simulink model "sgMdl_ResistorEmulation"  (R2024b)
settings: Solver=FixedStepAuto  StartTime=0.0  StopTime=inf  RelTol=1e-3  EnableMultiTasking=on
libraries: speedgoatlib_PIL x1, simulink x1
Description:
  | Resistor Emulation
settings Model: ModifiedByFormat=Speedgoat  SimulationMode=external  ExtModeTrigDuration=100000  Creator=Speedgoat  LastModifiedBy=Speedgoat
settings SolverCC: ConcurrentTasks=on  AlgebraicLoopSolver=TrustRegion  PositivePriorityOrder=on  InsertRTBMode=Never (minimum delay)
settings DataIOCC: SaveFormat=Array  SaveState=on  SignalLoggingName=logsOut
settings OptimizationCC: BlockReduction=off  BooleanDataType=off  OptimizeBlockIOStorage=off  BufferReuse=off  ReuseModelBlockBuffer=off  GlobalBufferReuse=off  ExpressionFolding=off  LocalBlockOutputs=off  InitFltsAndDblsToZero=on  OptimizeDataStoreBuffers=off  BusAssignmentInplaceUpdate=off
settings DebuggingCC: SaveWithParameterizedLinksMsg=none  UnderspecifiedInitializationDetection=Classic  MergeDetectMultiDrivingBlocksExec=none  CheckExecutionContextPreStartOutputMsg=on  SignalResolutionControl=TryResolveAllWithWarning  TasksWithSamePriorityMsg=none  UnconnectedInputMsg=warning  UnconnectedOutputMsg=warning  UnconnectedLineMsg=warning  SFUnexpectedBacktrackingDiag=warning  SFNoUnconditionalDefaultTransitionDiag=warning  SFExecutionAtInitializationDiag=none  ArithmeticOperatorsInVariantConditions=warning
settings HardwareCC: ProdBitPerLong=64  ProdLongLongMode=on  ProdHWDeviceType=Intel->x86-64 (Linux 64)
settings ModelReferenceCC: EnableRefExpFcnMdlSchedulingChecks=on  PropagateSignalLabelsOutOfModel=off
settings SFSimCC: SimUseLocalCustomCode=off  SimTargetLang=C++
settings RTWCC: Description=Speedgoat Real-Time Target Machine  SystemTargetFile=speedgoat.tlc  TemplateMakefile=slrealtime_default_tmf  PostCodeGenCommand=sg.model.build.makeCfg(bdroot, buildInfo);  RTWUseLocalCustomCode=off  Toolchain=Simulink Real-Time Toolchain  BuildConfiguration=Faster Runs  TargetLang=C++  GPUComputeCapability=3.5  DLArmComputeVersion=19.05
settings CodeAppCC: StateflowObjectComments=on
settings SimulinkRealTimeTargetCC: SubcomponentCodeInterfacePackaging=Reusable function  MATLABClassNameForMDSCustomization=Simulink.SoftwareTarget.GRTCustomization  InstructionSetFMA=off  LogToMDFFile=off  SLRTFileLogMaxRuns=10  UseGCCFastMath=on
settings ConfigComp: CovMetricSettings=dw  CovSaveCumulativeToWorkspaceVar=on  CovSaveSingleToWorkspaceVar=on  CovExternalEMLEnable=off  CovSFcnEnable=off  CovBoundaryAbsTol=1.0e-5

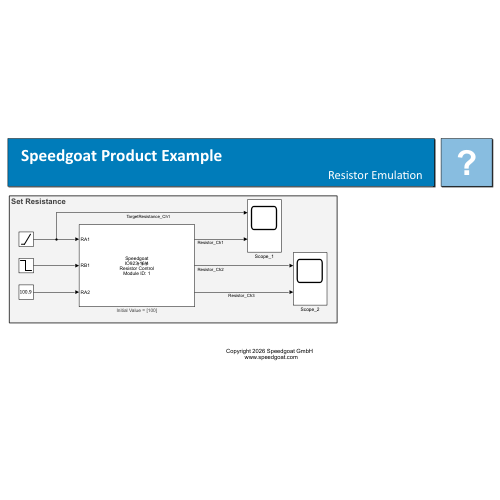
[thumbnail: Simulink's stored preview of the top-level diagram]
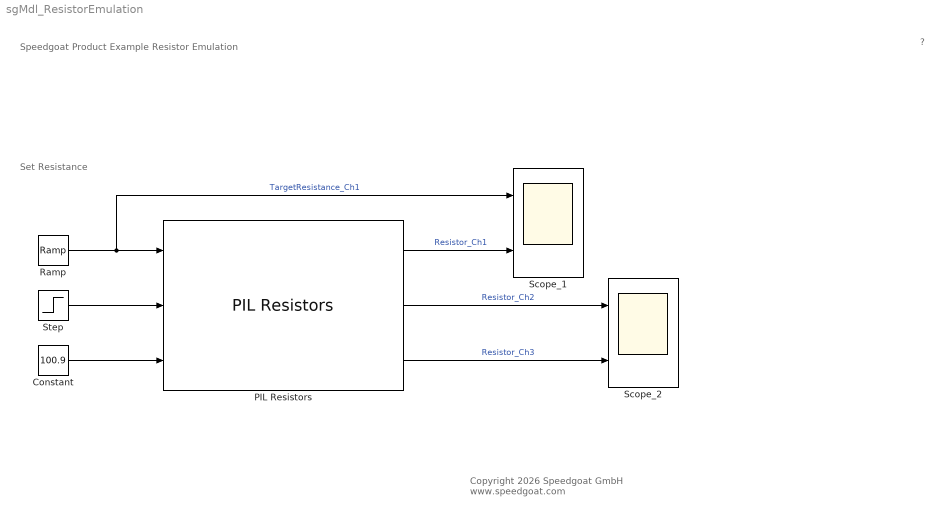
== system sgMdl_ResistorEmulation ==
  note: Set Resistance
  note: Speedgoat Product Example
      | Resistor Emulation
  note: ?
  note: Copyright 2026 Speedgoat GmbH
      |  www.speedgoat.com
  Constant : Constant  Value=100.9  OutDataTypeStr=Inherit: Inherit via back propagation  SampleTime=0.1
  PIL Resistors : speedgoatlib_PIL/PIL Resistors  id=1  card_type=IO921-12/10 (high density resistor simulation)  channel_vector=[1,2,3]  init_vector=[100]  reset_vector=[1]  show_output=on  ts=-1  slot=-1  VendorID=0  SubVendorID=0  DeviceID=0  SubDeviceID=0  category=1  NumCh=0  MinR=0  MaxR=0  bits=0  SupportsShort=0  SupportsOpen=0
      settings: AttributesFormatString=Initial Value = %<init_vector>  SourceProductName=Simulink Real-Time: Speedgoat I/O Blockset
  Ramp : simulink/Sources/Ramp  slope=1  start=2  InitialOutput=100
  Scope_1 : Scope  NumInputPorts=2
  Scope_2 : Scope  NumInputPorts=2
  Step : Step  Time=5  Before=100  After=0  SampleTime=0.1
  wires:
  PIL Resistors/3 -> Scope_2/2  "Resistor_Ch3"
  Constant/1 -> PIL Resistors/3
  Ramp/1 -> Scope_1/1, PIL Resistors/1  "TargetResistance_Ch1"
  PIL Resistors/1 -> Scope_1/2  "Resistor_Ch1"
  Step/1 -> PIL Resistors/2
  PIL Resistors/2 -> Scope_2/1  "Resistor_Ch2"
